simulink model "aerosonde_windup_model"  (R2018b)
settings: Solver=VariableStepAuto  StartTime=0.0  StopTime=t_final  MaxStep=deltaTMax  RelTol=1e-3
values from neighbouring files (symbols this model uses):
  KD_moment = 0    [aerosonde_windup.m]
  KD_thrust = .2    (= 0.2)    [aerosonde_windup.m]
  KI_moment = .40202*.01848    (= 0.0074293296)    [aerosonde_windup.m]
  KI_thrust = 0    [aerosonde_windup.m]
  KP_moment = .402002    (= 0.402002)    [aerosonde_windup.m]
  KP_thrust = 1    [aerosonde_windup.m]
  switchTime = 600    [aerosonde_windup.m]
  waypointRadius = 100    [aerosonde_windup.m]
  xILimitMoment = 0.05    [aerosonde_windup.m]
undefined symbols (not defined in the file or in its folder): GEOMETRY, xILimitThrust
libraries: PlanarVehicle x4, UWAerospaceBlockset_Controllers x3, UWControlsBlockset x2, aerolibanimutils x1
settings Model: Creator=Christopher  LastModifiedBy=Christopher
settings SimscapeCC: EditingMode=Restricted

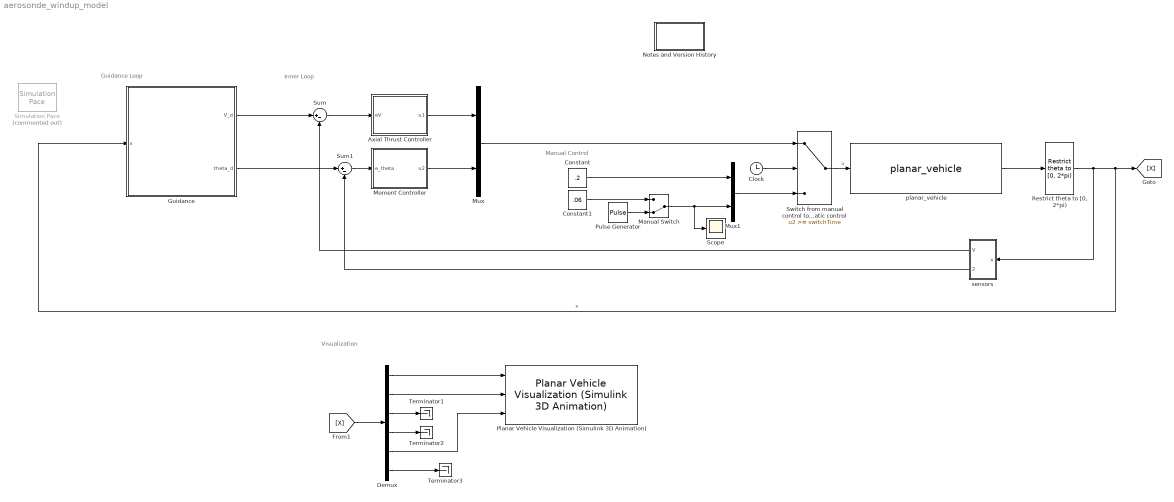
== system aerosonde_windup_model ==
  note: Manual Control
  note: Visualization
  note: Guidance Loop
  note: Inner Loop
  Axial Thrust Controller : Subsystem
  Clock : Clock
  Constant : Constant  Value=.2
  Constant1 : Constant  Value=.06
  Demux : Demux  Outputs=6
  Guidance : Subsystem
  Manual Switch : ManualSwitch  CurrentSetting=0
  Moment Controller : Subsystem
  Mux : Mux  Inputs=2
  Mux1 : Mux  Inputs=2
  Notes and Version History : Subsystem
  Planar Vehicle Visualization (Simulink 3D Animation) : PlanarVehicle/Planar Vehicle Visualization (Simulink 3D Animation)  T_animate=1
  Pulse Generator : DiscretePulseGenerator  PulseType=Time based  Period=100  PulseWidth=4.7
  "Restrict theta to [0, 2*pi)" : PlanarVehicle/Restrict theta to [0, 2*pi)  SystemSampleTime=-1
  Scope : Scope
  Simulation Pace : aerolibanimutils/Simulation Pace  Commented=on  SimulationPace=30  SleepMode=Auto  OutputPaceError=off  SampleTime=1/30
  Sum : Sum  Inputs=|+-
  Sum1 : Sum  Inputs=|+-
  Switch from manual control to automatic control : Switch  Threshold=switchTime
  Terminator1 : Terminator
  Terminator2 : Terminator
  Terminator3 : Terminator
  planar_vehicle : PlanarVehicle/planar_vehicle  m=GEOMETRY.mass  Ib=GEOMETRY.Ib  Fmax=PROPULSION.Fmax  Mmax=PROPULSION.Mmax  x0=SIMULATION.X_0  CT=ENVIRONMENT.CT  CR=ENVIRONMENT.CR
  sensors : Subsystem
  wires:
  Axial Thrust Controller/1(u1) -> Mux/1
  Moment Controller/1(u2) -> Mux/2
  sensors/2(theta) -> Sum1/2
  sensors/1(V) -> Sum/2
  Sum/1 -> Axial Thrust Controller/1(eV)
  Sum1/1 -> Moment Controller/1(e_theta)
  [X] -> Demux/1
  Demux/1 -> Planar Vehicle Visualization (Simulink 3D Animation)/1
  Demux/2 -> Planar Vehicle Visualization (Simulink 3D Animation)/2
  Demux/3 -> Terminator1/1
  Demux/4 -> Terminator2/1
  Demux/6 -> Terminator3/1
  Demux/5 -> Planar Vehicle Visualization (Simulink 3D Animation)/3
  "Restrict theta to [0, 2*pi)"/1 -> Guidance/1(x), [X], sensors/1(x)  "x"
  Guidance/1(V_d) -> Sum/1
  Guidance/2(theta_d) -> Sum1/1
  Switch from manual control to automatic control/1 -> planar_vehicle/1  "u"
  Constant/1 -> Mux1/1
  Manual Switch/1 -> Scope/1, Mux1/2
  Clock/1 -> Switch from manual control to automatic control/2
  Mux/1 -> Switch from manual control to automatic control/1
  Mux1/1 -> Switch from manual control to automatic control/3
  planar_vehicle/1 -> "Restrict theta to [0, 2*pi)"/1
  Constant1/1 -> Manual Switch/1
  Pulse Generator/1 -> Manual Switch/2

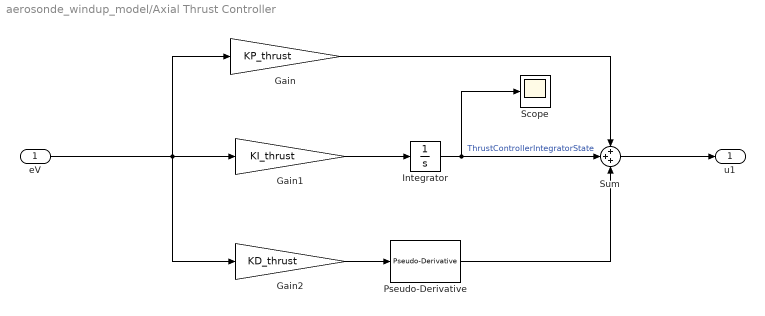
== system aerosonde_windup_model/Axial Thrust Controller ==
  eV : Inport
  Gain : Gain  Gain=KP_thrust
  Gain1 : Gain  Gain=KI_thrust
  Gain2 : Gain  Gain=KD_thrust
  Integrator : Integrator  UpperSaturationLimit=xILimitThrust  LowerSaturationLimit=-xILimitThrust
  Pseudo-Derivative : UWControlsBlockset/Pseudo-Derivative  a=a_thrust
  Scope : Scope
  Sum : Sum  Inputs=+++
  u1 : Outport
  wires:
  eV/1 -> Gain2/1, Gain1/1, Gain/1
  Gain/1 -> Sum/1
  Integrator/1 -> Scope/1, Sum/2  "ThrustControllerIntegratorState"
  Gain1/1 -> Integrator/1
  Gain2/1 -> Pseudo-Derivative/1
  Sum/1 -> u1/1
  Pseudo-Derivative/1 -> Sum/3

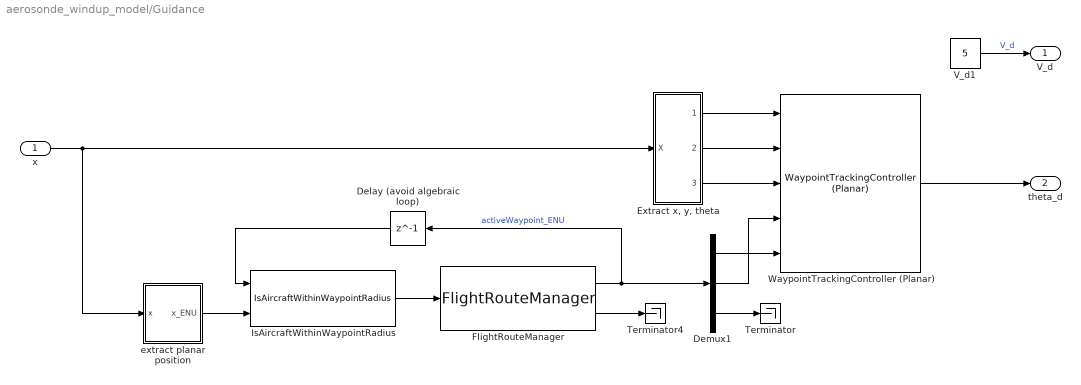
== system aerosonde_windup_model/Guidance ==
  x : Inport
  Delay (avoid algebraic loop) : Delay  DelayLength=1
  Demux1 : Demux  Outputs=3
  "Extract x, y, theta" : Subsystem
  FlightRouteManager : UWAerospaceBlockset_Controllers/FlightRouteManager  waypoints=flightRoute.Points  isClosedRoute=off
  IsAircraftWithinWaypointRadius : UWAerospaceBlockset_Controllers/IsAircraftWithinWaypointRadius  R=waypointRadius
  Terminator : Terminator
  Terminator4 : Terminator
  V_d1 : Constant  Value=5
  WaypointTrackingController (Planar) : UWAerospaceBlockset_Controllers/WaypointTrackingController (Planar)
  extract planar position : Subsystem
  V_d : Outport
  theta_d : Outport  Port=2
  wires:
  x/1 -> "Extract x, y, theta"/1(X), extract planar position/1(x)
  extract planar position/1(x_ENU) -> IsAircraftWithinWaypointRadius/2
  "Extract x, y, theta"/1(y = PN) -> WaypointTrackingController (Planar)/1
  FlightRouteManager/2 -> Terminator4/1
  FlightRouteManager/1 -> Delay (avoid algebraic loop)/1, Demux1/1  "activeWaypoint_ENU"
  Demux1/1 -> WaypointTrackingController (Planar)/5
  Demux1/3 -> Terminator/1
  IsAircraftWithinWaypointRadius/1 -> FlightRouteManager/1
  Delay (avoid algebraic loop)/1 -> IsAircraftWithinWaypointRadius/1
  Demux1/2 -> WaypointTrackingController (Planar)/4
  "Extract x, y, theta"/3(theta) -> WaypointTrackingController (Planar)/3
  "Extract x, y, theta"/2(x = PE) -> WaypointTrackingController (Planar)/2
  V_d1/1 -> V_d/1  "V_d"
  WaypointTrackingController (Planar)/1 -> theta_d/1

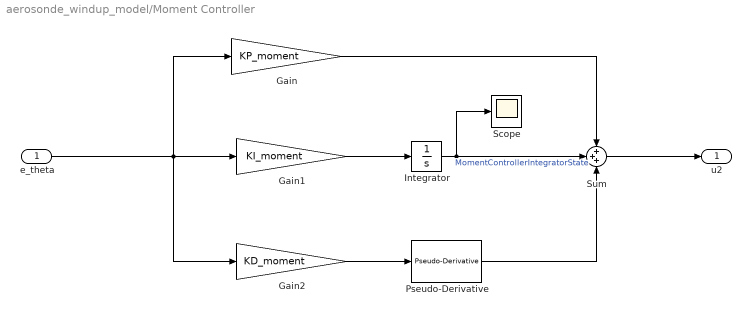
== system aerosonde_windup_model/Moment Controller ==
  e_theta : Inport
  Gain : Gain  Gain=KP_moment
  Gain1 : Gain  Gain=KI_moment
  Gain2 : Gain  Gain=KD_moment
  Integrator : Integrator  LimitOutput=on  UpperSaturationLimit=xILimitMoment  LowerSaturationLimit=-xILimitMoment
  Pseudo-Derivative : UWControlsBlockset/Pseudo-Derivative  a=a_moment
  Scope : Scope
  Sum : Sum  Inputs=+++
  u2 : Outport
  wires:
  Sum/1 -> u2/1
  Gain2/1 -> Pseudo-Derivative/1
  Gain1/1 -> Integrator/1
  Integrator/1 -> Scope/1, Sum/2  "MomentControllerIntegratorState"
  Gain/1 -> Sum/1
  e_theta/1 -> Gain/1, Gain1/1, Gain2/1
  Pseudo-Derivative/1 -> Sum/3

== system aerosonde_windup_model/Notes and Version History ==
  note: Version History
      | 05/02/21: Created from final project p2
  note: Version History
      | 05/02/21: Created from final project p2
      | 05/12/21: Updated to isolate integrator anti-windup limits

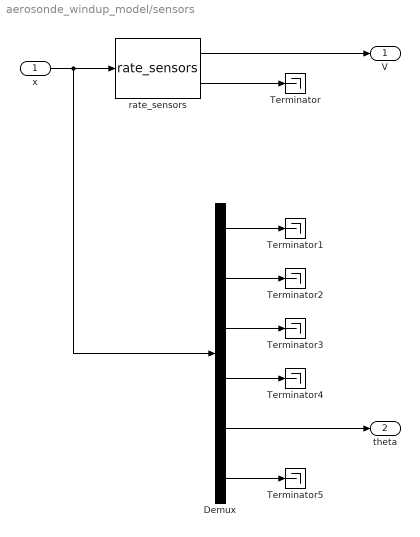
== system aerosonde_windup_model/sensors ==
  x : Inport
  Demux : Demux  Outputs=6
  Terminator{,1..5} (6 alike) : Terminator
  rate_sensors : PlanarVehicle/rate_sensors
  V : Outport
  theta : Outport  Port=2
  wires:
  x/1 -> Demux/1, rate_sensors/1
  rate_sensors/1 -> V/1
  Demux/5 -> theta/1
  rate_sensors/2 -> Terminator/1
  Demux/1 -> Terminator1/1
  Demux/2 -> Terminator2/1
  Demux/3 -> Terminator3/1
  Demux/4 -> Terminator4/1
  Demux/6 -> Terminator5/1

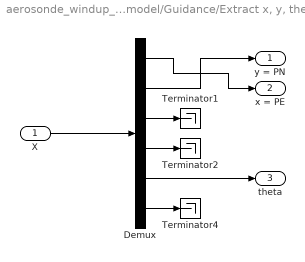
== system aerosonde_windup_model/Guidance/Extract x, y, theta ==
  X : Inport
  Demux : Demux  Outputs=6
  Terminator1 : Terminator
  Terminator2 : Terminator
  Terminator4 : Terminator
  y = PN : Outport
  x = PE : Outport  Port=2
  theta : Outport  Port=3
  wires:
  Demux/5 -> theta/1
  Demux/4 -> Terminator2/1
  Demux/3 -> Terminator1/1
  Demux/6 -> Terminator4/1
  X/1 -> Demux/1
  Demux/2 -> y = PN/1
  Demux/1 -> x = PE/1

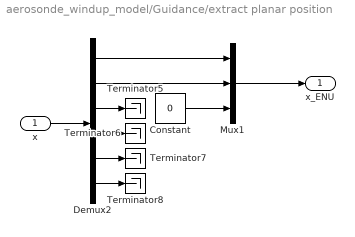
== system aerosonde_windup_model/Guidance/extract planar position ==
  x : Inport
  Constant : Constant  Value=0
  Demux2 : Demux  Outputs=6
  Mux1 : Mux  Inputs=3
  Terminator{5..8} (4 alike) : Terminator
  x_ENU : Outport
  wires:
  Demux2/4 -> Terminator6/1
  Mux1/1 -> x_ENU/1
  Demux2/3 -> Terminator5/1
  x/1 -> Demux2/1
  Constant/1 -> Mux1/3
  Demux2/2 -> Mux1/2
  Demux2/5 -> Terminator7/1
  Demux2/6 -> Terminator8/1
  Demux2/1 -> Mux1/1
